simulink model "lqg_d1"  (R2022a)
settings: Solver=VariableStepAuto  StartTime=0.0  StopTime=200  RelTol=1e-3
values from neighbouring files (symbols this model uses):
  Ad = sysd.a    [LQG_2by2_sim.m]
  Bd = sysd.b    [LQG_2by2_sim.m]
  K = (4-3*rho+q)./(8+10*rho+2*q)    [kalman_example.m]
undefined symbols (not defined in the file or in its folder): Cd, Kfilter, L, Ts, var_Te, var_v1, var_v2, var_va
settings Model: Creator=lplal  LastModifiedBy=Ccm

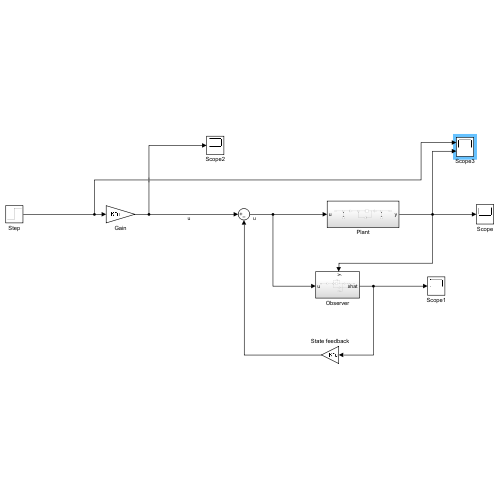
[thumbnail: Simulink's stored preview of the top-level diagram]
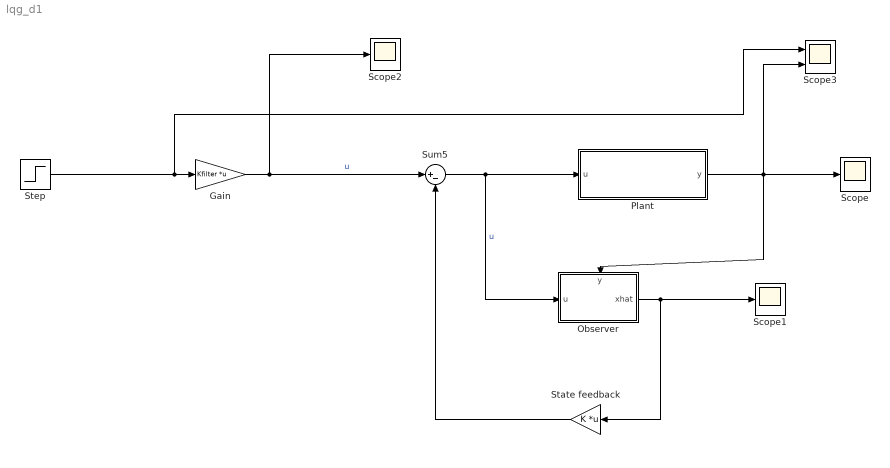
== system lqg_d1 ==
  Gain : Gain  Gain=Kfilter  Multiplication=Matrix(K*u)
  Observer : Subsystem
      settings: PortSchema="{\"entries\":[{\"content\":{\"sides\":[{\"content\":{\"connectorIds\":[\"In1\"]},\"type\":\"ConnectorPlacement.EquallySpacedRectSide\",\"uuid\":\"f4ae0740-89bf-4035-96e8-743ce40d8411\"},{\"content\":{\"connectorIds\":[\"Out1\"],\"side\":\"RIGHT\"},\"type\":\"ConnectorPlacement.EquallySpacedRectSide\",\"uuid\":\"278b155b-d02c-463a-b092-758e224a1d04\"},{\"content\":{\"connectorIds\":[\"In2\"],\"side\":\"TOP\"},\"type\":\"ConnectorPlacement.EquallySpacedRectSide\",\"uuid\":\"ed877ab8-76bc-4310-a07b-e9394956a7e0\"}]},\"type\":\"ConnectorPlacement.EquallySpacedConnector\",\"uuid\":\"8efaa953-734e-4e39-94c8-005649f57eca\"}],\"packageUris\":[\"http://schema.mathworks.com/mf0/Connector/R2020b\"],\"version\":\"1.0\"}"
  Plant : Subsystem
  Scope : Scope
  Scope1 : Scope
  Scope2 : Scope
  Scope3 : Scope  NumInputPorts=2
  State feedback : Gain  Gain=K  Multiplication=Matrix(K*u)
  Step : Step  Time=5  Before=10  After=100  SampleTime=0
  Sum5 : Sum  Inputs=|+-
  wires:
  Sum5/1 -> Observer/1(u), Plant/1(u)  "u"
  State feedback/1 -> Sum5/2
  Observer/1(xhat) -> State feedback/1, Scope1/1
  Plant/1(y) -> Scope3/2, Scope/1, Observer/2(y)
  Gain/1 -> Scope2/1, Sum5/1  "u"
  Step/1 -> Scope3/1, Gain/1

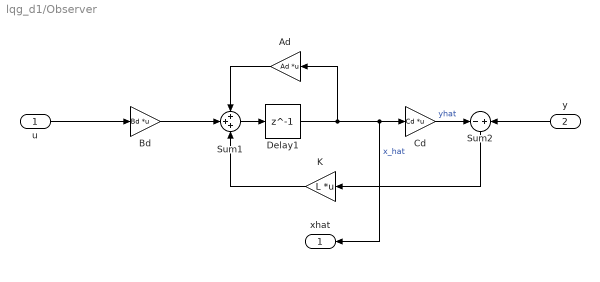
== system lqg_d1/Observer ==
  u : Inport
  y : Inport  Port=2
  Ad : Gain  Gain=Ad  Multiplication=Matrix(K*u)
  Bd : Gain  Gain=Bd  Multiplication=Matrix(K*u)
  Cd : Gain  Gain=Cd  Multiplication=Matrix(K*u)
  Delay1 : Delay  DelayLength=1
  K : Gain  Gain=L  Multiplication=Matrix(K*u)
  Sum1 : Sum  Inputs=+++
  Sum2 : Sum  Inputs=-|+
  xhat : Outport
  wires:
  Ad/1 -> Sum1/1
  Sum1/1 -> Delay1/1
  Sum2/1 -> K/1
  u/1 -> Bd/1
  Bd/1 -> Sum1/2
  y/1 -> Sum2/2
  K/1 -> Sum1/3
  Delay1/1 -> Ad/1, xhat/1, Cd/1  "x_hat"
  Cd/1 -> Sum2/1  "yhat"

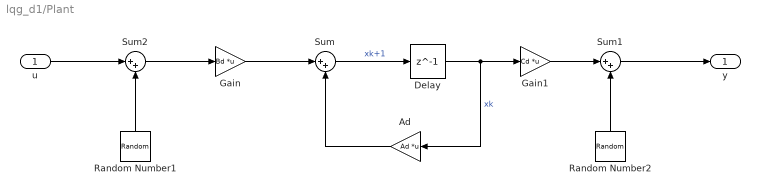
== system lqg_d1/Plant ==
  u : Inport
  Ad : Gain  Gain=Ad  Multiplication=Matrix(K*u)
  Delay : Delay  DelayLength=1  InitialCondition=0
  Gain : Gain  Gain=Bd  Multiplication=Matrix(K*u)
  Gain1 : Gain  Gain=Cd  Multiplication=Matrix(K*u)
  Random Number1 : RandomNumber  Variance=[var_va,var_Te]  SampleTime=Ts
  Random Number2 : RandomNumber  Variance=[var_v1,var_v2]  SampleTime=Ts
  Sum : Sum  Inputs=|++
  Sum1 : Sum  Inputs=|++
  Sum2 : Sum  Inputs=|++
  y : Outport
  wires:
  Sum2/1 -> Gain/1
  Sum1/1 -> y/1
  Sum/1 -> Delay/1  "xk+1"
  Delay/1 -> Ad/1, Gain1/1  "xk"
  Random Number2/1 -> Sum1/2
  Random Number1/1 -> Sum2/2
  u/1 -> Sum2/1
  Gain/1 -> Sum/1
  Gain1/1 -> Sum1/1
  Ad/1 -> Sum/2
